simulink model "atwood"  (R2024b)
settings: Solver=ode45  StartTime=0.0  StopTime=50  MaxStep=2^-5  RelTol=1^-3
libraries: simulink x2
settings Model: Creator=zv53855  LastModifiedBy=zv53855

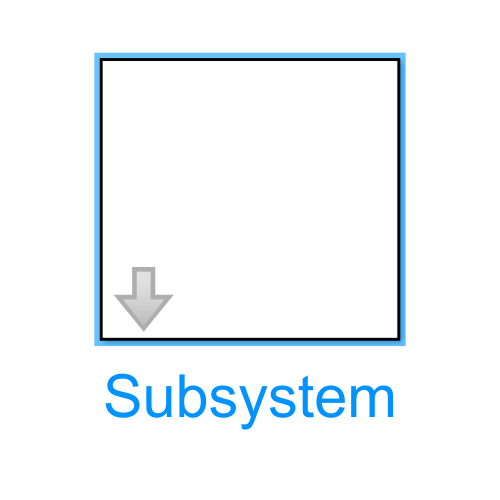
[thumbnail: Simulink's stored preview of the top-level diagram]
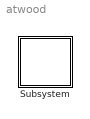
== system atwood ==
  Subsystem : Subsystem  mask{g=9.81, m1=0.5, m2=0.9, M=1, R=0.001, r0=1, theta0=120*pi/180}
      mask prompts: g "earth gravity"; m1 "pendulum mass"; m2 "load mass"; M "block math"; R "block r"; r0 "r(0)"; theta0 "theta(0)"

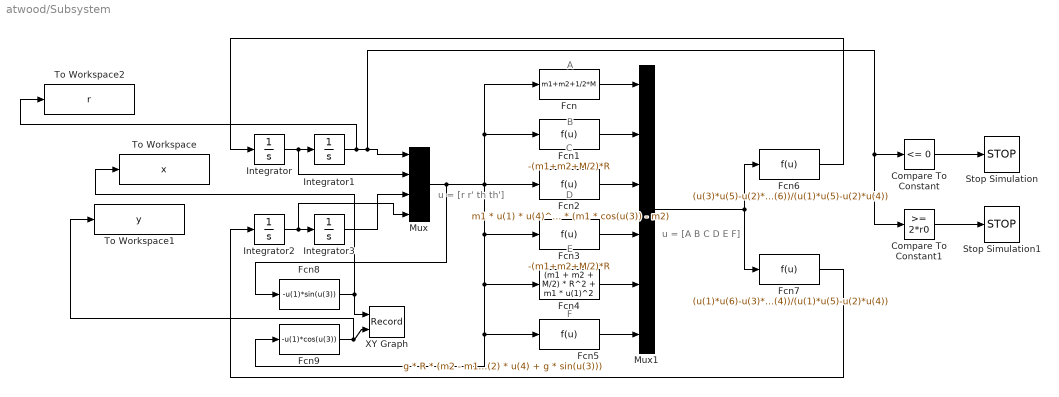
== system atwood/Subsystem ==
  note: u = [A B C D E F]
  note: F
  note: A
  note: u = [r r' th th']
  note: B
  note: C
  note: D
  note: E
  Compare To Constant : simulink/Logic and Bit Operations/Compare To Constant  relop=<=  const=0  OutDataTypeStr=boolean
  Compare To Constant1 : simulink/Logic and Bit Operations/Compare To Constant  relop=>=  const=2*r0  OutDataTypeStr=boolean
  Fcn : Fcn  Expr=m1+m2+1/2*M
  Fcn1 : Fcn  Expr=-(m1+m2+M/2)*R
  Fcn2 : Fcn  Expr=m1 * u(1) * u(4)^2 + g * (m1 * cos(u(3)) - m2)
  Fcn3 : Fcn  Expr=-(m1+m2+M/2)*R
  Fcn4 : Fcn  Expr=(m1 + m2 + M/2) * R^2 + m1 * u(1)^2
  Fcn5 : Fcn  Expr=g * R * (m2 - m1 * cos(u(3))) - m1 * u(1) * (2 * u(2) * u(4) + g * sin(u(3)))
  Fcn6 : Fcn  Expr=(u(3)*u(5)-u(2)*u(6))/(u(1)*u(5)-u(2)*u(4))
  Fcn7 : Fcn  Expr=(u(1)*u(6)-u(3)*u(4))/(u(1)*u(5)-u(2)*u(4))
  Fcn8 : Fcn  Expr=-u(1)*sin(u(3))
  Fcn9 : Fcn  Expr=-u(1)*cos(u(3))
  Integrator : Integrator
  Integrator1 : Integrator  InitialCondition=r0
  Integrator2 : Integrator
  Integrator3 : Integrator  InitialCondition=theta0
  Mux : Mux
  Mux1 : Mux  Inputs=6
  Stop Simulation : Stop
  Stop Simulation1 : Stop
  To Workspace : ToWorkspace  VariableName=x  SampleTime=-1
  To Workspace1 : ToWorkspace  VariableName=y  SampleTime=-1
  To Workspace2 : ToWorkspace  VariableName=r  SampleTime=-1
  XY Graph : Record  FileSettingsInternal="{\"entries\":[{\"content\":{\"excelSettings\":{\"content\":{},\"type\":\"Streamout.ExcelSettings\"}},\"type\":\"Streamout.FileSettingStorage\",\"uuid\":\"\"}],\"packageUris\":[\"http:\\/\\/schema.mathworks.com\\/mf0\\/streamout_blocks\\/R2020a\"],\"version\":\"1.0\"}"  Layout=[1 1]  SignalsInternal="{\"entries\":[{\"content\":{\"signals\":[{\"content\":{\"blockPath\":[],\"dimensions\":[1],\"domain\":\"\",\"lineColor\":\"#a2142f\",\"plots\":[ 1 ],\"port\":1,\"sid\":[\"\"],\"signalID\":1,\"signalName\":\"Fcn8\"},\"type\":\"RecordBlkView.Signal\",\"uuid\":\"\"},{\"content\":{\"blockPath\":[],\"dimensions\":[1],\"domain\":\"\",\"lineColor\":\"#139fff\",\"plots\":[ 1 ],\"port\":2,\"sid\":[\"\"],\"signalID\":2,\"signalName\":\"Fcn9\"},\"type\":\"RecordBlkView.Signal\",\"uuid\":\"\"}]},\"type\":\"RecordBlkView.InputSignals\",\"uuid\":\"\"}],\"packageUris\":[\"http:\\/\\/schema.mathworks.com\\/mf0\\/streamout_blocks\\/R2020a\"],\"version\":\"1.0\"}"  VisualizationBindings="{\"xyplotplugin\":{\"info\":[{\"series\":[{\"bindingParametersList\":[{\"parameter\":\"X-Axis\",\"signalID\":1,\"signalName\":\"Fcn8\"},{\"parameter\":\"Y-Axis\",\"signalID\":2,\"signalName\":\"Fcn9\"}],\"seriesID\":0}],\"subplotID\":1}]}}"  CompatibilityTag=XY
  wires:
  Integrator/1 -> Mux/2, Integrator1/1
  Integrator2/1 -> Mux/4, Integrator3/1
  Integrator1/1 -> To Workspace2/1, Compare To Constant1/1, Compare To Constant/1, Mux/1
  Integrator3/1 -> Mux/3
  Mux1/1 -> Fcn6/1, Fcn7/1
  Mux/1 -> Fcn8/1, Fcn9/1, Fcn5/1, Fcn4/1, Fcn3/1, Fcn1/1, Fcn/1, Fcn2/1
  Fcn/1 -> Mux1/1
  Fcn1/1 -> Mux1/2
  Fcn2/1 -> Mux1/3
  Fcn3/1 -> Mux1/4
  Fcn4/1 -> Mux1/5
  Fcn5/1 -> Mux1/6
  Fcn6/1 -> Integrator/1
  Fcn7/1 -> Integrator2/1
  Compare To Constant/1 -> Stop Simulation/1
  Compare To Constant1/1 -> Stop Simulation1/1
  Fcn8/1 -> XY Graph/1, To Workspace/1
  Fcn9/1 -> To Workspace1/1, XY Graph/2
